simulink model "Control"  (R2025b)
settings: configuration reference "code" (kept outside this file)
undefined symbols (not defined in the file or in its folder): D1, P
settings Model: DataDictionary=test.sldd  Creator=rpumpo  LastModifiedBy=rpumpo
settings ConfigSetRef: SourceName=code

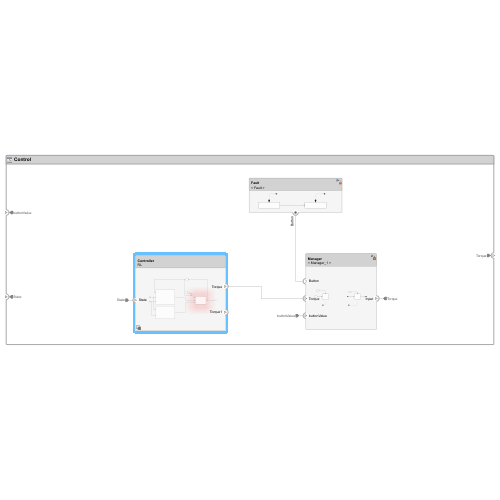
[thumbnail: Simulink's stored preview of the top-level diagram]
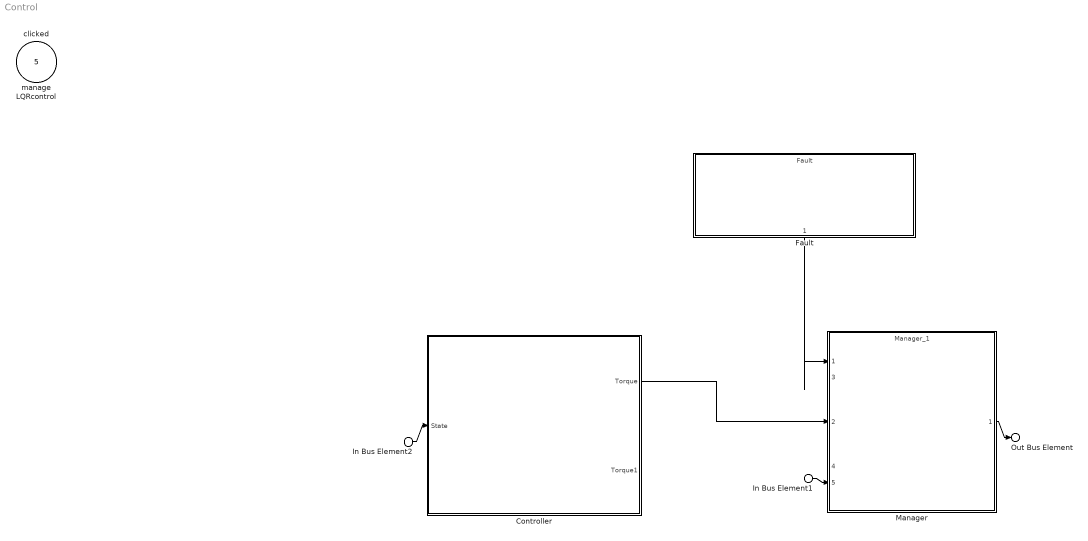
== system Control ==
  In Bus Element1 : Inport  PortName=buttonValue
  In Bus Element2 : Inport  Port=2  PortName=State
  manage : Inport  Port=3  OutputFunctionCall=on
  clicked : Inport  Port=4  OutputFunctionCall=on
  LQRcontrol : Inport  Port=5  OutputFunctionCall=on
  Controller : Subsystem  Variant=on  VariantControlMode=label  LabelModeActiveChoice=RL
      settings: PortSchema="{\"entries\":[{\"content\":{\"headerSize\":38,\"margin\":15,\"minimumSpacing\":25,\"sides\":[{\"content\":{\"connectorIds\":[\"In1\"]},\"type\":\"ConnectorPlacement.EquallySpacedRectSide\",\"uuid\":\"863a0b16-e36b-44d6-9477-1468a80c696d\"},{\"content\":{\"connectorIds\":[\"Out1\",\"Out2\"],\"side\":\"RIGHT\"},\"type\":\"ConnectorPlacement.EquallySpacedRectSide\",\"uuid\":\"ac9067ee-3fe6-46b1-b4d3-b466d54413ae\"},{\"content\":{\"side\":\"TOP\"},\"type\":\"ConnectorPlacement.EquallySpacedRectSide\",\"uuid\":\"d4aa2d7a-4362-47d2-9788-fc41168b683c\"},{\"content\":{\"side\":\"HIDDEN\"},\"type\":\"ConnectorPlacement.EquallySpacedRectSide\",\"uuid\":\"60b27dcf-8fa0-4a89-bb01-87fe99356072\"}]},\"type\":\"ConnectorPlacement.EquallySpacedConnector\",\"uuid\":\"884a1123-87f2-4a92-8ca9-5d4169531818\"}],\"packageUris\":[\"http://schema.mathworks.com/mf0/Connector/R2020b\"],\"version\":\"1.0\"}"
  Fault : ModelReference  ModelNameDialog=Fault  SimulationMode=Normal  ScheduleRates=on  ModelReferenceVersion=1.21
      settings: PortSchema="{\"entries\":[{\"content\":{\"headerSize\":38,\"margin\":15,\"minimumSpacing\":25,\"sides\":[{\"content\":{},\"type\":\"ConnectorPlacement.EquallySpacedRectSide\",\"uuid\":\"863a0b16-e36b-44d6-9477-1468a80c696d\"},{\"content\":{\"side\":\"RIGHT\"},\"type\":\"ConnectorPlacement.EquallySpacedRectSide\",\"uuid\":\"ac9067ee-3fe6-46b1-b4d3-b466d54413ae\"},{\"content\":{\"side\":\"TOP\"},\"type\":\"ConnectorPlacement.EquallySpacedRectSide\",\"uuid\":\"d4aa2d7a-4362-47d2-9788-fc41168b683c\"},{\"content\":{\"connectorIds\":[\"Out1\"],\"side\":\"BOTTOM\"},\"type\":\"ConnectorPlacement.EquallySpacedRectSide\",\"uuid\":\"0123640a-2603-4642-b39e-a5ff4c76992d\"}]},\"type\":\"ConnectorPlacement.EquallySpacedConnector\",\"uuid\":\"884a1123-87f2-4a92-8ca9-5d4169531818\"}],\"packageUris\":[\"http://schema.mathworks.com/mf0/Connector/R2020b\"],\"version\":\"1.0\"}"
  Manager : ModelReference  ModelNameDialog=Manager_1  SimulationMode=Normal  ScheduleRates=on  ModelReferenceVersion=1.16
      settings: PortSchema="{\"entries\":[{\"content\":{\"headerSize\":38,\"margin\":15,\"minimumSpacing\":25,\"sides\":[{\"content\":{\"connectorIds\":[\"In1\",\"In2\",\"In5\"]},\"type\":\"ConnectorPlacement.EquallySpacedRectSide\",\"uuid\":\"c8b0d3d9-bc3c-4342-81a6-a8c7ff56dd35\"},{\"content\":{\"connectorIds\":[\"Out1\"],\"side\":\"RIGHT\"},\"type\":\"ConnectorPlacement.EquallySpacedRectSide\",\"uuid\":\"d4831bcc-b3df-49cd-9384-d58cd33334b8\"},{\"content\":{\"side\":\"TOP\"},\"type\":\"ConnectorPlacement.EquallySpacedRectSide\",\"uuid\":\"1cd8d703-8026-4c12-b737-e2eb28763fcc\"},{\"content\":{\"connectorIds\":[\"In3\",\"In4\"],\"side\":\"HIDDEN\"},\"type\":\"ConnectorPlacement.EquallySpacedRectSide\",\"uuid\":\"1189461b-4f41-4411-bd17-a372f5f5f715\"}]},\"type\":\"ConnectorPlacement.EquallySpacedConnector\",\"uuid\":\"3c898837-2af3-4ac4-a686-c1110b7b9353\"}],\"packageUris\":[\"http://schema.mathworks.com/mf0/Connector/R2020b\"],\"version\":\"1.0\"}"
  Out Bus Element : Outport  PortName=Torque
  wires:
  Manager/1 -> Out Bus Element/1
  Fault/1 -> Manager/1
  In Bus Element1/1 -> Manager/5
  In Bus Element2/1 -> Controller/1(State)
  Controller/1(Torque) -> Manager/2

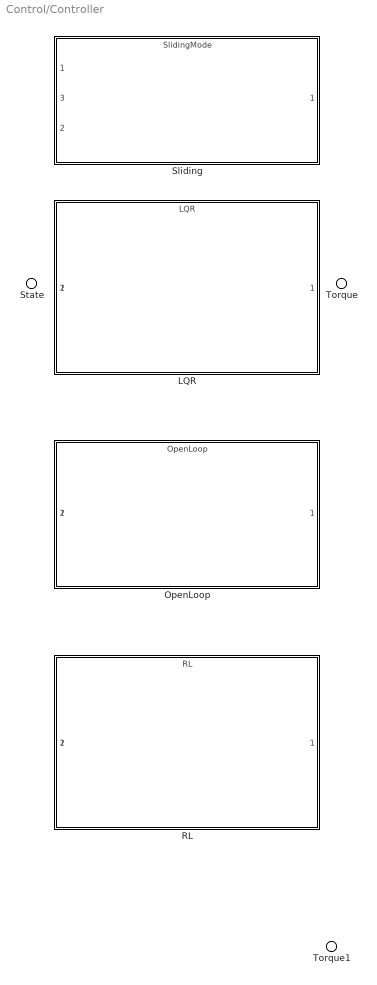
== system Control/Controller ==
  State : Inport
  LQR : ModelReference  ModelNameDialog=LQR  SimulationMode=Normal  ScheduleRates=on  CachedPortDiscreteRates=[-1]  VariantControl=LQR  ModelReferenceVersion=1.16
      settings: PortSchema="{\"entries\":[{\"content\":{\"headerSize\":38,\"margin\":15,\"minimumSpacing\":25,\"sides\":[{\"content\":{\"connectorIds\":[\"In1\"]},\"type\":\"ConnectorPlacement.EquallySpacedRectSide\",\"uuid\":\"863a0b16-e36b-44d6-9477-1468a80c696d\"},{\"content\":{\"connectorIds\":[\"Out1\"],\"side\":\"RIGHT\"},\"type\":\"ConnectorPlacement.EquallySpacedRectSide\",\"uuid\":\"ac9067ee-3fe6-46b1-b4d3-b466d54413ae\"},{\"content\":{\"side\":\"TOP\"},\"type\":\"ConnectorPlacement.EquallySpacedRectSide\",\"uuid\":\"d4aa2d7a-4362-47d2-9788-fc41168b683c\"},{\"content\":{\"connectorIds\":[\"In2\"],\"side\":\"HIDDEN\"},\"type\":\"ConnectorPlacement.EquallySpacedRectSide\",\"uuid\":\"60b27dcf-8fa0-4a89-bb01-87fe99356072\"}]},\"type\":\"ConnectorPlacement.EquallySpacedConnector\",\"uuid\":\"884a1123-87f2-4a92-8ca9-5d4169531818\"}],\"packageUris\":[\"http://schema.mathworks.com/mf0/Connector/R2020b\"],\"version\":\"1.0\"}"
  OpenLoop : ModelReference  ModelNameDialog=OpenLoop  SimulationMode=Normal  ScheduleRates=on  CachedPortDiscreteRates=[0.001]  ModelEventPortInfo=P:D1[0.001][0][0]  VariantControl=OpenLoop  ModelReferenceVersion=1.4
      settings: PortSchema="{\"entries\":[{\"content\":{\"headerSize\":38,\"margin\":15,\"minimumSpacing\":25,\"sides\":[{\"content\":{\"connectorIds\":[\"In1\"]},\"type\":\"ConnectorPlacement.EquallySpacedRectSide\",\"uuid\":\"e3850213-7836-4a76-9138-db9561f2dfa3\"},{\"content\":{\"connectorIds\":[\"Out1\"],\"side\":\"RIGHT\"},\"type\":\"ConnectorPlacement.EquallySpacedRectSide\",\"uuid\":\"0376d83e-b2c6-47e1-ac72-ef48c291ef7a\"},{\"content\":{\"side\":\"TOP\"},\"type\":\"ConnectorPlacement.EquallySpacedRectSide\",\"uuid\":\"0ca152af-581b-44cc-8c1a-1940fec58944\"},{\"content\":{\"connectorIds\":[\"In2\"],\"side\":\"HIDDEN\"},\"type\":\"ConnectorPlacement.EquallySpacedRectSide\",\"uuid\":\"837c145c-6633-4f3c-aecb-1a10664e2aa0\"}]},\"type\":\"ConnectorPlacement.EquallySpacedConnector\",\"uuid\":\"7f3a45e2-30ac-43d0-98f3-5299d75cc4ed\"}],\"packageUris\":[\"http://schema.mathworks.com/mf0/Connector/R2020b\"],\"version\":\"1.0\"}"
  RL : ModelReference  ModelNameDialog=RL.slx  SimulationMode=Normal  ScheduleRates=on  CachedPortDiscreteRates=[-1]  ModelEventPortInfo=P:D1[-1][0][0]  VariantControl=RL  ModelReferenceVersion=1.8
      settings: PortSchema="{\"entries\":[{\"content\":{\"headerSize\":38,\"margin\":15,\"minimumSpacing\":25,\"sides\":[{\"content\":{\"connectorIds\":[\"In1\"]},\"type\":\"ConnectorPlacement.EquallySpacedRectSide\",\"uuid\":\"863a0b16-e36b-44d6-9477-1468a80c696d\"},{\"content\":{\"connectorIds\":[\"Out1\"],\"side\":\"RIGHT\"},\"type\":\"ConnectorPlacement.EquallySpacedRectSide\",\"uuid\":\"ac9067ee-3fe6-46b1-b4d3-b466d54413ae\"},{\"content\":{\"side\":\"TOP\"},\"type\":\"ConnectorPlacement.EquallySpacedRectSide\",\"uuid\":\"d4aa2d7a-4362-47d2-9788-fc41168b683c\"},{\"content\":{\"connectorIds\":[\"In2\"],\"side\":\"HIDDEN\"},\"type\":\"ConnectorPlacement.EquallySpacedRectSide\",\"uuid\":\"60b27dcf-8fa0-4a89-bb01-87fe99356072\"}]},\"type\":\"ConnectorPlacement.EquallySpacedConnector\",\"uuid\":\"884a1123-87f2-4a92-8ca9-5d4169531818\"}],\"packageUris\":[\"http://schema.mathworks.com/mf0/Connector/R2020b\"],\"version\":\"1.0\"}"
  Sliding : ModelReference  ModelNameDialog=SlidingMode.slx  SimulationMode=Normal  ScheduleRates=on  CachedPortDiscreteRates=[-1]  VariantControl=Sliding  ModelReferenceVersion=1.19
      settings: PortSchema="{\"entries\":[{\"content\":{\"headerSize\":38,\"margin\":15,\"minimumSpacing\":25,\"sides\":[{\"content\":{\"connectorIds\":[\"In1\",\"In2\"]},\"type\":\"ConnectorPlacement.EquallySpacedRectSide\",\"uuid\":\"eab79fa7-634d-4a94-a9ba-d7989084414f\"},{\"content\":{\"connectorIds\":[\"Out1\"],\"side\":\"RIGHT\"},\"type\":\"ConnectorPlacement.EquallySpacedRectSide\",\"uuid\":\"7ef4c35f-e29a-4703-a19f-7e0690d8ee25\"},{\"content\":{\"side\":\"TOP\"},\"type\":\"ConnectorPlacement.EquallySpacedRectSide\",\"uuid\":\"022f6fec-93f0-44b1-8207-af5780452d6e\"},{\"content\":{\"connectorIds\":[\"In3\"],\"side\":\"HIDDEN\"},\"type\":\"ConnectorPlacement.EquallySpacedRectSide\",\"uuid\":\"950fcd50-b445-4bba-bee8-5e79db60bfe0\"}]},\"type\":\"ConnectorPlacement.EquallySpacedConnector\",\"uuid\":\"0b578510-fead-4794-81f6-8cc0e72415a8\"}],\"packageUris\":[\"http://schema.mathworks.com/mf0/Connector/R2020b\"],\"version\":\"1.0\"}"
  Torque : Outport
  Torque1 : Outport  Port=2
